simulink model "vvc1phase_simpower"  (Simulink 10.2)
settings: Solver=ode3  StartTime=0.0  StopTime=0.5  FixedStep=.00000005  MaxStep=.0000001  RelTol=1e-3  EnableMultiTasking=on
libraries: powerlib x32, simulink x11
(part 2 of 2)

== system vvc1phase_simpower/SensorSigProc_Sinc3_N512_38p4us ==
  note: Sinc3, N=512, 20MHz to 39kHz, settling time = 3*512*0.05e-6=76us, delay=38.4us
  Input : Inport
  Discrete Integrator : DiscreteFilter  Denominator=[1 -1]
  Discrete Integrator1 : DiscreteFilter  Denominator=[1 -1]
  Discrete Integrator2 : DiscreteFilter  Denominator=[1 -1]
  Discrete differentiator : DiscreteFilter  Numerator=[1 -1]  Denominator=[1]
  Discrete differentiator1 : DiscreteFilter  Numerator=[1 -1]  Denominator=[1]
  Discrete differentiator2 : DiscreteFilter  Numerator=[1 -1]  Denominator=[1]
  Gain : Gain  Gain=1/512
  Gain1 : Gain  Gain=1/512
  Gain2 : Gain  Gain=1/512
  Rate Transition : RateTransition
  Zero-Order Hold : ZeroOrderHold  SampleTime=512*0.05e-6
  Zero-Order Hold2 : ZeroOrderHold  SampleTime=.00000005
  Output : Outport
  wires:
  Rate Transition/1 -> Zero-Order Hold2/1
  Zero-Order Hold2/1 -> Output/1
  Discrete differentiator2/1 -> Gain2/1
  Discrete differentiator1/1 -> Gain1/1
  Discrete differentiator/1 -> Gain/1
  Zero-Order Hold/1 -> Discrete differentiator/1
  Discrete Integrator2/1 -> Zero-Order Hold/1
  Discrete Integrator1/1 -> Discrete Integrator2/1
  Discrete Integrator/1 -> Discrete Integrator1/1
  Input/1 -> Discrete Integrator/1
  Gain/1 -> Discrete differentiator1/1
  Gain1/1 -> Discrete differentiator2/1
  Gain2/1 -> Rate Transition/1

== system vvc1phase_simpower/SensorSigProc_Sinc3_N512_38p4us1 ==
  note: Sinc3, N=512, 20MHz to 39kHz, settling time = 3*512*0.05e-6=76us, delay=38.4us
  Input : Inport
  Discrete Integrator : DiscreteFilter  Denominator=[1 -1]
  Discrete Integrator1 : DiscreteFilter  Denominator=[1 -1]
  Discrete Integrator2 : DiscreteFilter  Denominator=[1 -1]
  Discrete differentiator : DiscreteFilter  Numerator=[1 -1]  Denominator=[1]
  Discrete differentiator1 : DiscreteFilter  Numerator=[1 -1]  Denominator=[1]
  Discrete differentiator2 : DiscreteFilter  Numerator=[1 -1]  Denominator=[1]
  Gain : Gain  Gain=1/512
  Gain1 : Gain  Gain=1/512
  Gain2 : Gain  Gain=1/512
  Rate Transition : RateTransition
  Zero-Order Hold : ZeroOrderHold  SampleTime=512*0.05e-6
  Zero-Order Hold2 : ZeroOrderHold  SampleTime=.00000005
  Output : Outport
  wires:
  Gain2/1 -> Rate Transition/1
  Gain1/1 -> Discrete differentiator2/1
  Gain/1 -> Discrete differentiator1/1
  Input/1 -> Discrete Integrator/1
  Discrete Integrator/1 -> Discrete Integrator1/1
  Discrete Integrator1/1 -> Discrete Integrator2/1
  Discrete Integrator2/1 -> Zero-Order Hold/1
  Zero-Order Hold/1 -> Discrete differentiator/1
  Discrete differentiator/1 -> Gain/1
  Discrete differentiator1/1 -> Gain1/1
  Discrete differentiator2/1 -> Gain2/1
  Zero-Order Hold2/1 -> Output/1
  Rate Transition/1 -> Zero-Order Hold2/1

== system vvc1phase_simpower/SensorSigProc_Sinc3_N8_0p6us2_UNSTABLE_USE_INT16_VERSION ==
  note: Sinc3, N=8, 20MHz to 2.5MHz, settling time = 3*8*0.05e-6=1.2us, delay=0.6us
  Input : Inport
  Discrete Integrator : DiscreteFilter  Denominator=[1 -1]
  Discrete Integrator1 : DiscreteFilter  Denominator=[1 -1]
  Discrete Integrator2 : DiscreteFilter  Denominator=[1 -1]
  Discrete differentiator : DiscreteFilter  Numerator=[1 -1]  Denominator=[1]
  Discrete differentiator1 : DiscreteFilter  Numerator=[1 -1]  Denominator=[1]
  Discrete differentiator2 : DiscreteFilter  Numerator=[1 -1]  Denominator=[1]
  Gain : Gain  Gain=1/8
  Gain1 : Gain  Gain=1/8
  Gain2 : Gain  Gain=1/8
  Rate Transition : RateTransition
  Zero-Order Hold : ZeroOrderHold  SampleTime=8*0.05e-6
  Zero-Order Hold2 : ZeroOrderHold  SampleTime=.00000005
  Output : Outport
  wires:
  Gain2/1 -> Rate Transition/1
  Gain1/1 -> Discrete differentiator2/1
  Gain/1 -> Discrete differentiator1/1
  Input/1 -> Discrete Integrator/1
  Discrete Integrator/1 -> Discrete Integrator1/1
  Discrete Integrator1/1 -> Discrete Integrator2/1
  Discrete Integrator2/1 -> Zero-Order Hold/1
  Zero-Order Hold/1 -> Discrete differentiator/1
  Discrete differentiator/1 -> Gain/1
  Discrete differentiator1/1 -> Gain1/1
  Discrete differentiator2/1 -> Gain2/1
  Zero-Order Hold2/1 -> Output/1
  Rate Transition/1 -> Zero-Order Hold2/1

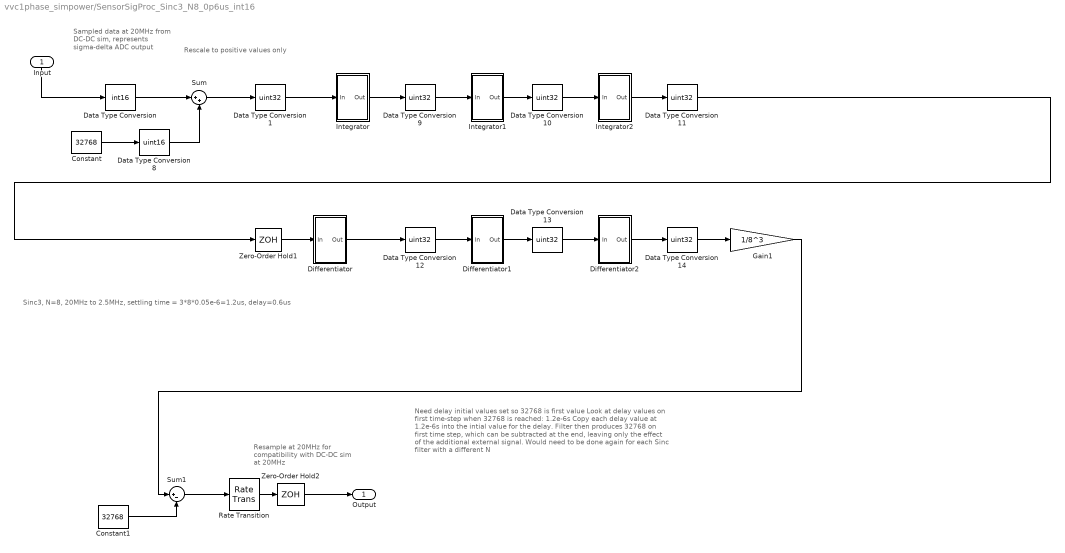
== system vvc1phase_simpower/SensorSigProc_Sinc3_N8_0p6us_int16 ==
  note: Resample at 20MHz
      | for compatibility with
      | DC-DC sim at 20MHz
  note: Need delay initial values set so 32768 is first value
      | Look at delay values on first time-step when 32768 is reached: 1.2e-6s
      | Copy each delay value at 1.2e-6s into the intial value for the delay.
      | Filter then produces 32768 on first time step, which can be
      | subtracted at the end, leaving only the effect of the
      | additional external signal.
      |
      | Would need to be done again for each Sinc filter with a different N
  note: Rescale to positive values only
  note: Sinc3, N=8, 20MHz to 2.5MHz, settling time = 3*8*0.05e-6=1.2us, delay=0.6us
  note: Sampled data at 20MHz
      | from DC-DC sim, represents
      | sigma-delta ADC output
  Input : Inport
  Constant : Constant  Value=32768
  Constant1 : Constant  Value=32768
  Data Type Conversion : DataTypeConversion  OutDataTypeStr=int16
  Data Type Conversion{1,9..14} (7 alike) : DataTypeConversion  OutDataTypeStr=uint32
  Data Type Conversion8 : DataTypeConversion  OutDataTypeStr=uint16
  Differentiator : Subsystem
  Differentiator1 : Subsystem
  Differentiator2 : Subsystem
  Gain1 : Gain  Gain=1/8^3
  Integrator : Subsystem
  Integrator1 : Subsystem
  Integrator2 : Subsystem
  Rate Transition : RateTransition
  Sum : Sum  Inputs=|++
  Sum1 : Sum  Inputs=|+-
  Zero-Order Hold1 : ZeroOrderHold  SampleTime=8*0.05e-6
  Zero-Order Hold2 : ZeroOrderHold  SampleTime=.00000005
  Output : Outport
  wires:
  Rate Transition/1 -> Zero-Order Hold2/1
  Zero-Order Hold2/1 -> Output/1
  Input/1 -> Data Type Conversion/1
  Data Type Conversion/1 -> Sum/1
  Constant/1 -> Data Type Conversion8/1
  Sum/1 -> Data Type Conversion1/1
  Constant1/1 -> Sum1/2
  Sum1/1 -> Rate Transition/1
  Data Type Conversion8/1 -> Sum/2
  Data Type Conversion1/1 -> Integrator/1(In)
  Integrator/1(Out) -> Data Type Conversion9/1
  Differentiator/1(Out) -> Data Type Conversion12/1
  Data Type Conversion12/1 -> Differentiator1/1(In)
  Differentiator1/1(Out) -> Data Type Conversion13/1
  Data Type Conversion13/1 -> Differentiator2/1(In)
  Differentiator2/1(Out) -> Data Type Conversion14/1
  Data Type Conversion14/1 -> Gain1/1
  Gain1/1 -> Sum1/1
  Zero-Order Hold1/1 -> Differentiator/1(In)
  Integrator1/1(Out) -> Data Type Conversion10/1
  Data Type Conversion10/1 -> Integrator2/1(In)
  Integrator2/1(Out) -> Data Type Conversion11/1
  Data Type Conversion9/1 -> Integrator1/1(In)
  Data Type Conversion11/1 -> Zero-Order Hold1/1

== system vvc1phase_simpower/counter  ==
  gate signal : Inport
  Add : Sum
  Data Type Conversion : DataTypeConversion  OutDataTypeStr=int32
  Delay1 : Delay  DelayLength=1  InitialCondition=0
  Delay2 : Delay  DelayLength=1  InitialCondition=0
  Logical Operator2 : Logic  Operator=XOR  AllPortsSameDT=off  OutDataTypeStr=boolean
  count : Outport
  wires:
  Add/1 -> count/1, Delay1/1
  Delay2/1 -> Logical Operator2/2
  Logical Operator2/1 -> Data Type Conversion/1
  Delay1/1 -> Add/1
  gate signal/1 -> Delay2/1, Logical Operator2/1
  Data Type Conversion/1 -> Add/2

== system vvc1phase_simpower/Controller10kHzHysteresisVPIBen/Subsystem ==
  current error : Inport
  upper bound : Inport  Port=2
  lower bound : Inport  Port=3
  Delay : Delay  DelayLength=1  InitialCondition=0
  Index Vector : MultiPortSwitch  DataPortOrder=Zero-based contiguous  Inputs=2  zeroidx=on
  Logical Operator : Logic  Operator=NOT  AllPortsSameDT=off  OutDataTypeStr=boolean
  Logical Operator1 : Logic  Operator=OR  AllPortsSameDT=off  OutDataTypeStr=boolean
  Relational Operator : RelationalOperator  OutDataTypeStr=boolean  RndMeth=Nearest
  Relational Operator1 : RelationalOperator  Operator=<=  OutDataTypeStr=boolean  RndMeth=Nearest
  GateDriveHi_Bool : Outport
  GateDriveLo_Bool : Outport  Port=2
  wires:
  current error/1 -> Relational Operator1/1, Relational Operator/1
  upper bound/1 -> Relational Operator/2
  lower bound/1 -> Relational Operator1/2
  Logical Operator1/1 -> Index Vector/1
  Relational Operator1/1 -> Logical Operator1/2, Index Vector/3
  Delay/1 -> Index Vector/2
  Relational Operator/1 -> Logical Operator1/1
  Logical Operator/1 -> GateDriveLo_Bool/1
  Index Vector/1 -> Delay/1, GateDriveHi_Bool/1, Logical Operator/1

== system vvc1phase_simpower/Controller10kHzHysteresisVPIMax/Subsystem ==
  current error : Inport
  upper bound : Inport  Port=2
  lower bound : Inport  Port=3
  Delay : Delay  DelayLength=1  InitialCondition=0
  Index Vector : MultiPortSwitch  DataPortOrder=Zero-based contiguous  Inputs=2  zeroidx=on
  Logical Operator : Logic  Operator=NOT  AllPortsSameDT=off  OutDataTypeStr=boolean
  Logical Operator1 : Logic  Operator=OR  AllPortsSameDT=off  OutDataTypeStr=boolean
  Relational Operator : RelationalOperator  OutDataTypeStr=boolean  RndMeth=Nearest
  Relational Operator1 : RelationalOperator  Operator=<=  OutDataTypeStr=boolean  RndMeth=Nearest
  GateDriveHi_Bool : Outport
  GateDriveLo_Bool : Outport  Port=2
  wires:
  Logical Operator/1 -> GateDriveLo_Bool/1
  Index Vector/1 -> Delay/1, Logical Operator/1, GateDriveHi_Bool/1
  Relational Operator/1 -> Logical Operator1/1
  Delay/1 -> Index Vector/2
  Relational Operator1/1 -> Index Vector/3, Logical Operator1/2
  Logical Operator1/1 -> Index Vector/1
  lower bound/1 -> Relational Operator1/2
  upper bound/1 -> Relational Operator/2
  current error/1 -> Relational Operator/1, Relational Operator1/1

== system vvc1phase_simpower/Controller50kHzHysteresisVPIBen/Subsystem ==
  current error : Inport
  upper bound : Inport  Port=2
  lower bound : Inport  Port=3
  Delay : Delay  DelayLength=1  InitialCondition=0
  Index Vector : MultiPortSwitch  DataPortOrder=Zero-based contiguous  Inputs=2  zeroidx=on
  Logical Operator : Logic  Operator=NOT  AllPortsSameDT=off  OutDataTypeStr=boolean
  Logical Operator1 : Logic  Operator=OR  AllPortsSameDT=off  OutDataTypeStr=boolean
  Relational Operator : RelationalOperator  OutDataTypeStr=boolean  RndMeth=Nearest
  Relational Operator1 : RelationalOperator  Operator=<=  OutDataTypeStr=boolean  RndMeth=Nearest
  GateDriveHi_Bool : Outport
  GateDriveLo_Bool : Outport  Port=2
  wires:
  Logical Operator/1 -> GateDriveLo_Bool/1
  Index Vector/1 -> Delay/1, Logical Operator/1, GateDriveHi_Bool/1
  Relational Operator/1 -> Logical Operator1/1
  Delay/1 -> Index Vector/2
  Relational Operator1/1 -> Index Vector/3, Logical Operator1/2
  Logical Operator1/1 -> Index Vector/1
  lower bound/1 -> Relational Operator1/2
  upper bound/1 -> Relational Operator/2
  current error/1 -> Relational Operator/1, Relational Operator1/1

== system vvc1phase_simpower/Controller50kHzHysteresisVPIMax/Subsystem ==
  current error : Inport
  upper bound : Inport  Port=2
  lower bound : Inport  Port=3
  Delay : Delay  DelayLength=1  InitialCondition=0
  Index Vector : MultiPortSwitch  DataPortOrder=Zero-based contiguous  Inputs=2  zeroidx=on
  Logical Operator : Logic  Operator=NOT  AllPortsSameDT=off  OutDataTypeStr=boolean
  Logical Operator1 : Logic  Operator=OR  AllPortsSameDT=off  OutDataTypeStr=boolean
  Relational Operator : RelationalOperator  OutDataTypeStr=boolean  RndMeth=Nearest
  Relational Operator1 : RelationalOperator  Operator=<=  OutDataTypeStr=boolean  RndMeth=Nearest
  GateDriveHi_Bool : Outport
  GateDriveLo_Bool : Outport  Port=2
  wires:
  current error/1 -> Relational Operator1/1, Relational Operator/1
  upper bound/1 -> Relational Operator/2
  lower bound/1 -> Relational Operator1/2
  Logical Operator1/1 -> Index Vector/1
  Relational Operator1/1 -> Logical Operator1/2, Index Vector/3
  Delay/1 -> Index Vector/2
  Relational Operator/1 -> Logical Operator1/1
  Index Vector/1 -> GateDriveHi_Bool/1, Logical Operator/1, Delay/1
  Logical Operator/1 -> GateDriveLo_Bool/1

== system vvc1phase_simpower/SensorSigProc_Sinc3_N8_0p6us_int16/Differentiator ==
  In : Inport
  Delay : Delay  DelayLength=1  InitialCondition=31752192
  Sum2 : Sum  Inputs=|+-
  Out : Outport
  wires:
  Sum2/1 -> Out/1
  In/1 -> Delay/1, Sum2/1
  Delay/1 -> Sum2/2

== system vvc1phase_simpower/SensorSigProc_Sinc3_N8_0p6us_int16/Differentiator1 ==
  In : Inport
  Delay : Delay  DelayLength=1  InitialCondition=26345472
  Display : Display
  Sum2 : Sum  Inputs=|+-
  Out : Outport
  wires:
  Delay/1 -> Display/1, Sum2/2
  In/1 -> Sum2/1, Delay/1
  Sum2/1 -> Out/1

== system vvc1phase_simpower/SensorSigProc_Sinc3_N8_0p6us_int16/Differentiator2 ==
  In : Inport
  Delay : Delay  DelayLength=1  InitialCondition=20971520
  Display : Display
  Sum2 : Sum  Inputs=|+-
  Out : Outport
  wires:
  Sum2/1 -> Out/1
  In/1 -> Delay/1, Sum2/1
  Delay/1 -> Display/1, Sum2/2

== system vvc1phase_simpower/SensorSigProc_Sinc3_N8_0p6us_int16/Integrator ==
  In : Inport
  Delay : Delay  DelayLength=1  InitialCondition=786432
  Sum2 : Sum  Inputs=|++
  Out : Outport
  wires:
  In/1 -> Sum2/1
  Sum2/1 -> Out/1, Delay/1
  Delay/1 -> Sum2/2

== system vvc1phase_simpower/SensorSigProc_Sinc3_N8_0p6us_int16/Integrator1 ==
  In : Inport
  Delay : Delay  DelayLength=1  InitialCondition=9830400
  Sum2 : Sum  Inputs=|++
  Out : Outport
  wires:
  Delay/1 -> Sum2/2
  Sum2/1 -> Delay/1, Out/1
  In/1 -> Sum2/1

== system vvc1phase_simpower/SensorSigProc_Sinc3_N8_0p6us_int16/Integrator2 ==
  In : Inport
  Delay : Delay  DelayLength=1  InitialCondition=85196800
  Sum2 : Sum  Inputs=|++
  Out : Outport
  wires:
  In/1 -> Sum2/1
  Sum2/1 -> Out/1, Delay/1
  Delay/1 -> Sum2/2
